simulink library "csu_kir_image_request_lib"  (R2015b)
settings: Solver=ode45  StartTime=0.0  StopTime=10.0  RelTol=1e-3
undefined symbols (not defined in the file): cam_kir_image_size, cam_kir_intrinsics
libraries: util_info_lib x2
settings Model: Creator=escrane  LastModifiedBy=jimkaidy
settings DataIOCC: SaveFormat=Array
settings DebuggingCC: UnderspecifiedInitializationDetection=Classic  MergeDetectMultiDrivingBlocksExec=none  SolverPrmCheckMsg=warning  StateNameClashWarn=warning
settings HardwareCC: ProdBitPerPointer=32  ProdLargestAtomicFloat=None  ProdIntDivRoundTo=Undefined  ProdEndianess=Unspecified  ProdWordSize=32  ProdHWDeviceType=32-bit Generic
settings GRTTargetCC: GeneratePreprocessorConditionals=Disable all
settings ConfigComp: CovModelRefEnable=Off  CovSFcnEnable=off

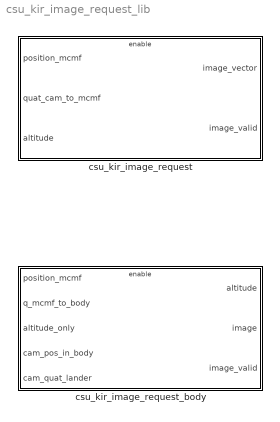
== system csu_kir_image_request_lib ==
  csu_kir_image_request : Subsystem  mask{size=cam_kir_image_size, intrinsics=cam_kir_intrinsics}
      mask prompts: size "Image Size [cols rows]"; intrinsics "Camera Intrinsics [f pixel_size]"
  csu_kir_image_request_body : Subsystem  mask{size=cam_kir_image_size, intrinsics=cam_kir_intrinsics}
      mask prompts: size "Image Size [cols rows]"; intrinsics "Camera Intrinsics [f pixel_size]"

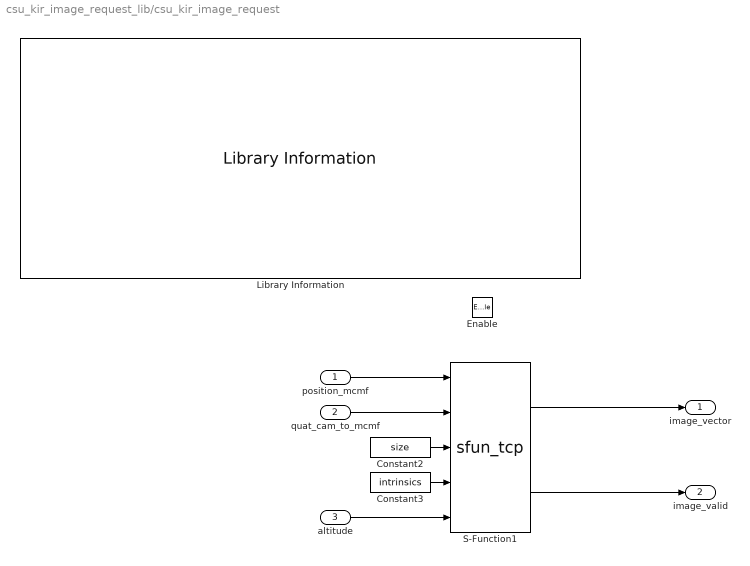
== system csu_kir_image_request_lib/csu_kir_image_request ==
  position_mcmf : Inport
  quat_cam_to_mcmf : Inport  Port=2
  altitude : Inport  Port=3
  Enable : EnablePort
  Constant2 : Constant  Value=size
  Constant3 : Constant  Value=intrinsics
  Library Information : util_info_lib/Library Information  owner='NONE'
  S-Function1 : S-Function  FunctionName=sfun_tcp  Parameters=192 168 1 12 5000  SFunctionDeploymentMode=off  EnableBusSupport=off
  image_vector : Outport
  image_valid : Outport  Port=2  InitialOutput=0
  wires:
  S-Function1/1 -> image_vector/1
  position_mcmf/1 -> S-Function1/1
  quat_cam_to_mcmf/1 -> S-Function1/2
  altitude/1 -> S-Function1/5
  Constant2/1 -> S-Function1/3
  Constant3/1 -> S-Function1/4
  S-Function1/2 -> image_valid/1

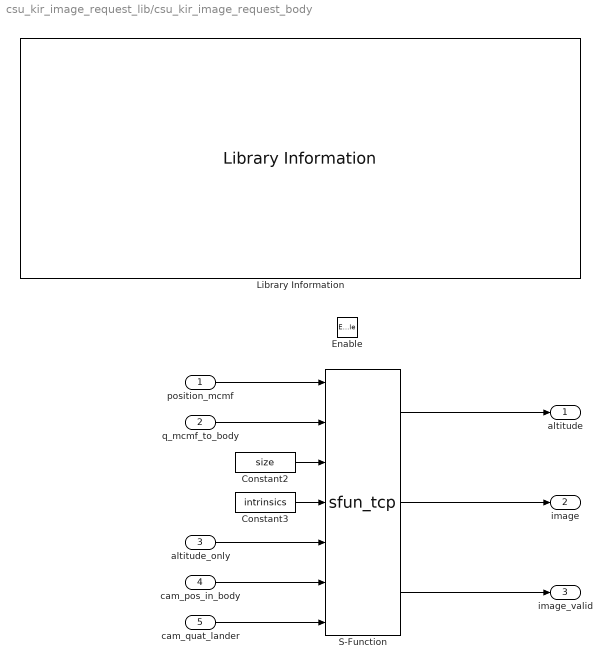
== system csu_kir_image_request_lib/csu_kir_image_request_body ==
  position_mcmf : Inport
  q_mcmf_to_body : Inport  Port=2
  altitude_only : Inport  Port=3
  cam_pos_in_body : Inport  Port=4
  cam_quat_lander : Inport  Port=5
  Enable : EnablePort
  Constant2 : Constant  Value=size
  Constant3 : Constant  Value=intrinsics
  Library Information : util_info_lib/Library Information  owner='NONE'
  S-Function : S-Function  FunctionName=sfun_tcp  Parameters=192 168 1 12 5000  SFunctionDeploymentMode=off  EnableBusSupport=off
  altitude : Outport
  image : Outport  Port=2  InitialOutput=0
  image_valid : Outport  Port=3  InitialOutput=0
  wires:
  S-Function/3 -> image_valid/1
  S-Function/1 -> altitude/1
  position_mcmf/1 -> S-Function/1
  q_mcmf_to_body/1 -> S-Function/2
  altitude_only/1 -> S-Function/5
  Constant2/1 -> S-Function/3
  Constant3/1 -> S-Function/4
  S-Function/2 -> image/1
  cam_pos_in_body/1 -> S-Function/6
  cam_quat_lander/1 -> S-Function/7
